simulink model "mix_fq_01"  (Simulink 8.6)
settings: Solver=VariableStepAuto  StartTime=1  StopTime=3  MaxStep=0.000001  RelTol=1e-3
values from neighbouring files (symbols this model uses):
  delay_1 = delay(1)    [environ.m]    (also in mix_fq_m.m = 0.014)
  delay_2 = delay(2)    [environ.m]    (also in mix_fq_m.m = 0.014)
  delay_3 = delay(3)    [environ.m]    (also in mix_fq_m.m = 0.014)
libraries: dsparch4 x6, commchan3 x3, commsynccomp2 x1, simulink x1
settings Model: Creator=my88899  LastModifiedBy=my88899
settings SolverCC: InitialStep=0.000001
settings DataIOCC: SaveFormat=Dataset  SignalLoggingSaveFormat=Dataset
settings OptimizationCC: ExpressionDepthLimit=128
settings DebuggingCC: UnderspecifiedInitializationDetection=Simplified  MergeDetectMultiDrivingBlocksExec=error  SolverPrmCheckMsg=none  FcnCallInpInsideContextMsg=EnableAllAsError  StateNameClashWarn=none
settings HardwareCC: ProdBitPerPointer=64  ProdLargestAtomicFloat=Float  ProdIntDivRoundTo=Zero  ProdEndianess=LittleEndian  ProdWordSize=64  ProdHWDeviceType=Intel->x86-64 (Windows64)
settings GRTTargetCC: GeneratePreprocessorConditionals=Use local settings  CombineOutputUpdateFcns=on  GRTInterface=off
settings ConfigComp: CovModelRefEnable=off
settings ConfigurationSet: Description=SimMechanics 2G

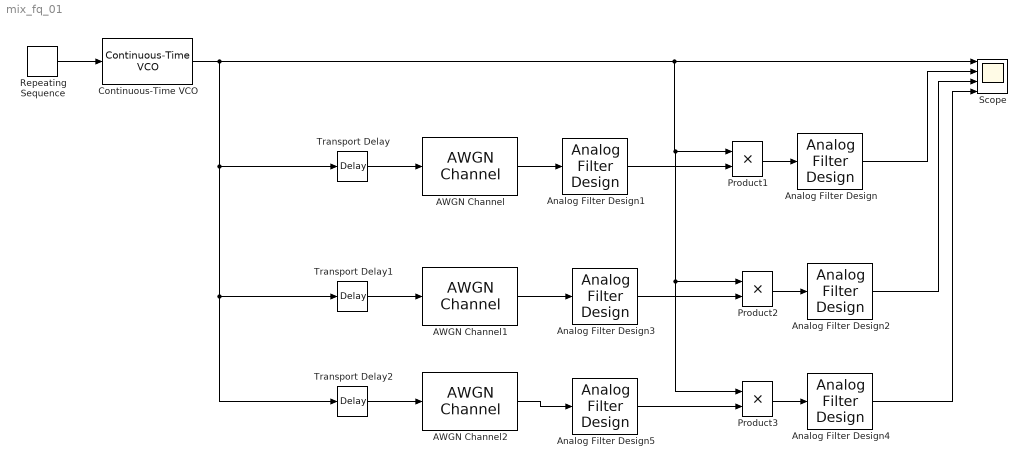
== system mix_fq_01 ==
  AWGN Channel : commchan3/AWGN Channel  InputProcessing=Columns as channels (frame based)  seed=67  noiseMode=Variance from mask  EbNodB=10  EsNodB=10  SNRdB=10  bitsPerSym=1  Ps=1  Tsym=1000000  variance=1
  AWGN Channel1 : commchan3/AWGN Channel  InputProcessing=Columns as channels (frame based)  seed=67  noiseMode=Variance from mask  EbNodB=10  EsNodB=10  SNRdB=10  bitsPerSym=1  Ps=1  Tsym=1000000  variance=1
  AWGN Channel2 : commchan3/AWGN Channel  InputProcessing=Columns as channels (frame based)  seed=67  noiseMode=Variance from mask  EbNodB=10  EsNodB=10  SNRdB=10  bitsPerSym=1  Ps=1  Tsym=1000000  variance=1
  Analog Filter Design : dsparch4/Analog Filter Design  method=Butterworth  filttype=Lowpass  N=12  Wlo=2*pi*20000  Whi=80  Rp=2  Rs=40
  Analog Filter Design1 : dsparch4/Analog Filter Design  method=Butterworth  filttype=Highpass  N=12  Wlo=2*pi*10000  Whi=80  Rp=2  Rs=40
  Analog Filter Design2 : dsparch4/Analog Filter Design  method=Butterworth  filttype=Lowpass  N=12  Wlo=2*pi*20000  Whi=80  Rp=2  Rs=40
  Analog Filter Design3 : dsparch4/Analog Filter Design  method=Butterworth  filttype=Highpass  N=12  Wlo=2*pi*10000  Whi=80  Rp=2  Rs=40
  Analog Filter Design4 : dsparch4/Analog Filter Design  method=Butterworth  filttype=Lowpass  N=12  Wlo=2*pi*20000  Whi=80  Rp=2  Rs=40
  Analog Filter Design5 : dsparch4/Analog Filter Design  method=Butterworth  filttype=Highpass  N=12  Wlo=2*pi*10000  Whi=80  Rp=2  Rs=40
  Continuous-Time VCO : commsynccomp2/Continuous-Time VCO  Ac=5  Fc=100000  Kc=10000  Ph=0
  Product1 : Product
  Product2 : Product
  Product3 : Product
  Repeating Sequence : simulink/Sources/Repeating Sequence  rep_seq_t=[0 1]  rep_seq_y=[0 10]
  Scope : Scope  NumInputPorts=4
  Transport Delay : TransportDelay  DelayTime=delay_1  BufferSize=3000000
  Transport Delay1 : TransportDelay  DelayTime=delay_2  BufferSize=3000000
  Transport Delay2 : TransportDelay  DelayTime=delay_3  BufferSize=3000000
  wires:
  Repeating Sequence/1 -> Continuous-Time VCO/1
  Analog Filter Design/1 -> Scope/2
  Product1/1 -> Analog Filter Design/1
  Transport Delay/1 -> AWGN Channel/1
  Analog Filter Design1/1 -> Product1/2
  AWGN Channel/1 -> Analog Filter Design1/1
  Transport Delay1/1 -> AWGN Channel1/1
  Transport Delay2/1 -> AWGN Channel2/1
  Analog Filter Design2/1 -> Scope/3
  Product2/1 -> Analog Filter Design2/1
  Analog Filter Design3/1 -> Product2/2
  AWGN Channel1/1 -> Analog Filter Design3/1
  Continuous-Time VCO/1 -> Product3/1, Product2/1, Product1/1, Scope/1, Transport Delay2/1, Transport Delay1/1, Transport Delay/1
  Analog Filter Design4/1 -> Scope/4
  Product3/1 -> Analog Filter Design4/1
  Analog Filter Design5/1 -> Product3/2
  AWGN Channel2/1 -> Analog Filter Design5/1
